simulink model "sf_fxptgf"  (Simulink 6.0)
settings: Solver=ode45  StartTime=0.0  StopTime=13  MaxStep=.1  RelTol=1e-3
settings Model: CovMetricSettings=dcmtr  Creator=The MathWorks Inc.  LastModifiedBy=batserve  ExtModeAutoUpdateStatusClock=off
settings DataIOCC: SignalLoggingName=sigsOut
settings DebuggingCC: CheckExecutionContextPreStartOutputMsg=on  CheckExecutionContextRuntimeOutputMsg=on  SolverPrmCheckMsg=none  ParameterOverflowMsg=warning
settings HardwareCC: TargetUnknown=on

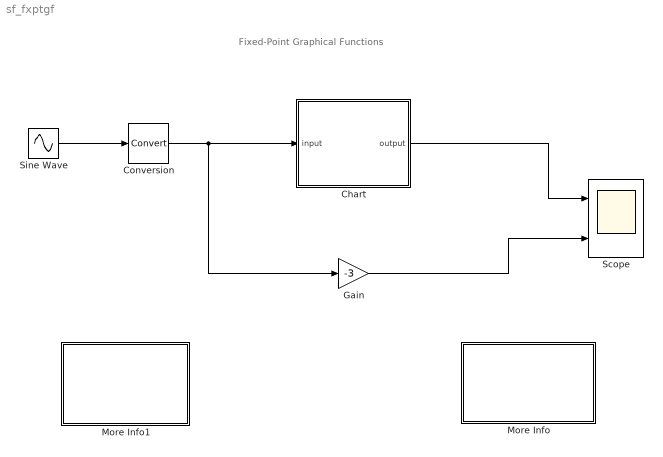
== system sf_fxptgf ==
  note: Fixed-Point Graphical Functions
  Chart : Stateflow chart  PropExecContextAcrossSSBoundary=on
  Conversion : DataTypeConversion  OutDataTypeMode=Specify via dialog  OutScaling=2^-4
  Gain : Gain  Gain=-3  SaturateOnIntegerOverflow=on
  More Info : Subsystem  PropExecContextAcrossSSBoundary=on
      mask Display: disp('Double click\nhere for\ninformation on\nthis demonstration')
  More Info1 : Subsystem  PropExecContextAcrossSSBoundary=on
      settings: OpenFcn=simcad(bdroot);
      mask Display: disp('Double click\nhere for\nSimulink\Stateflow\n Help')
  Scope : Scope  NumInputPorts=2
      settings: YMin=0~-4  YMax=3~4
  Sine Wave : Sin  SampleTime=0
  wires:
  Sine Wave/1 -> Conversion/1
  Chart/1(output) -> Scope/1
  Gain/1 -> Scope/2
  Conversion/1 -> Chart/1(input), Gain/1

== system sf_fxptgf/More Info ==
  note: Fixed-point data types can also be used as inputs to Graphical Functions within Stateflow. In this
      | demonstration, we provide a 16 bit signed input to the Stateflow chart from Simulink and send out
      | double. Within the chart, a graphical function uses takes the input and multiplies it by 3 if the value
      | is greater than or equal to zero or by -3 if the value is less than zero. The output is then converted
      | back to a double-precision float and sent to a scope block.
  note: Fixed-Point Graphical Functions

== system sf_fxptgf/More Info1 ==

== stateflow chart Chart ==
  state out = fixout(fixin) [function]
    (default) -> (junction 5)
    (junction 5) -> (junction 6) : [fixin>=0]{out=3*fixin;}
    (junction 5) -> (junction 7) : {out=-3*fixin;}
  (default) -> (junction 4) : {output=fixout(input);}
  data: fixin function_input fixpt; out function_output double; input input fixpt; output output double
